simulink model "REBEC2A_Remote"  (R2022b)
settings: Solver=VariableStepAuto  StartTime=0.0  StopTime=inf  FixedStep=0.001  RelTol=1e-3
InitFcn:
  | Remote = ihm_control;
  | import net.java.games.input.*;
StartFcn:
  | Throttle_Xbox = 'REBEC2A_Remote/Throttle_Xbox';
  | event_Throttle_Xbox = 'PostOutputs';
  | listener_Throttle_Xbox = @(app, event_Throttle_Xbox) updateGUI(Remote);
  | Throttle_Xbox_exec = add_exec_event_listener(Throttle_Xbox, event_Throttle_Xbox, listener_Throttle_Xbox);
  | 
  | Steering_Xbox = 'REBEC2A_Remote/Steering_Xbox';
  | event_Steering_Xbox = 'PostOutputs';
  | listener_Steering_Xbox = @(app, event_Steering_Xbox) updateGUI(Remote);
  | Steering_Xbox_exec = add_exec_event_listener(Steering_Xbox, event_Steering_Xbox, listener_Steering_Xbox);
  | 
  | Steering_IA = 'REBEC2A_Remote/Steering_IA';
  | event_Steering_IA = 'PostOutputs';
  | listener_Steering_IA = @(app, event_Steering_IA) updateGUI(Remote);
  | Steering_IA_exec = add_exec_event_listener(Steering_IA, event_Steering_IA, listener_Steering_IA);
  | 
  | Throttle_IA = 'REBEC2A_Remote/Throttle_IA';
  | event_Throttle_IA = 'PostOutputs';
  | listener_Throttle_IA = @(app, event_Throttle_IA) updateGUI(Remote);
  | Throttle_IA_exec = add_exec_event_listener(Throttle_IA, event_Throttle_IA, listener_Throttle_IA);
  | 
  | Steering_G920 = 'REBEC2A_Remote/Steering_G920';
  | event_Steering_G920 = 'PostOutputs';
  | listener_Steering_G920 = @(app, event_Steering_G920) updateGUI(Remote);
  | Steering_G920_exec = add_exec_event_listener(Steering_G920, event_Steering_G920, listener_Steering_G920);
  | 
  | Throttle_G920 = 'REBEC2A_Remote/Throttle_G920';
  | event_Throttle_G920 = 'PostOutputs';
  | listener_Throttle_G920 = @(app, event_Throttle_G920) updateGUI(Remote);
  | Throttle_G920_exec = add_exec_event_listener(Throttle_G920, event_Throttle_G920, listener_Throttle_G920);
  | 
  | ButtonA_G920 = 'REBEC2A_Remote/ButtonA_G920';
  | event_ButtonA_G920 = 'PostOutputs';
  | listener_ButtonA_G920 = @(app, event_ButtonA_G920) updateGUI(Remote);
  | ButtonA_G920_exec = add_exec_event_listener(ButtonA_G920, event_ButtonA_G920, listener_ButtonA_G920);
StopFcn:
  | close all force;
undefined symbols (not defined in the file or in its folder): DiscIntNeverNeededParam
libraries: simulink x2, vrlib x1
settings Model: SimulationMode=accelerator  Creator=Mathias Voigt  LastModifiedBy=Xen
settings SolverCC: AlgebraicLoopSolver=TrustRegion
settings DebuggingCC: UnconnectedInputMsg=warning  UnconnectedOutputMsg=warning  UnconnectedLineMsg=warning  SFMachineParentedDataDiag=warning
settings ModelReferenceCC: EnableRefExpFcnMdlSchedulingChecks=on
settings SFSimCC: CustomCodeUndefinedFunction=UseInterfaceOnly

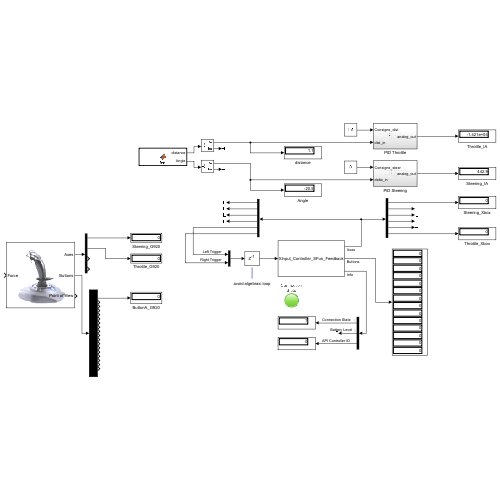
[thumbnail: Simulink's stored preview of the top-level diagram]
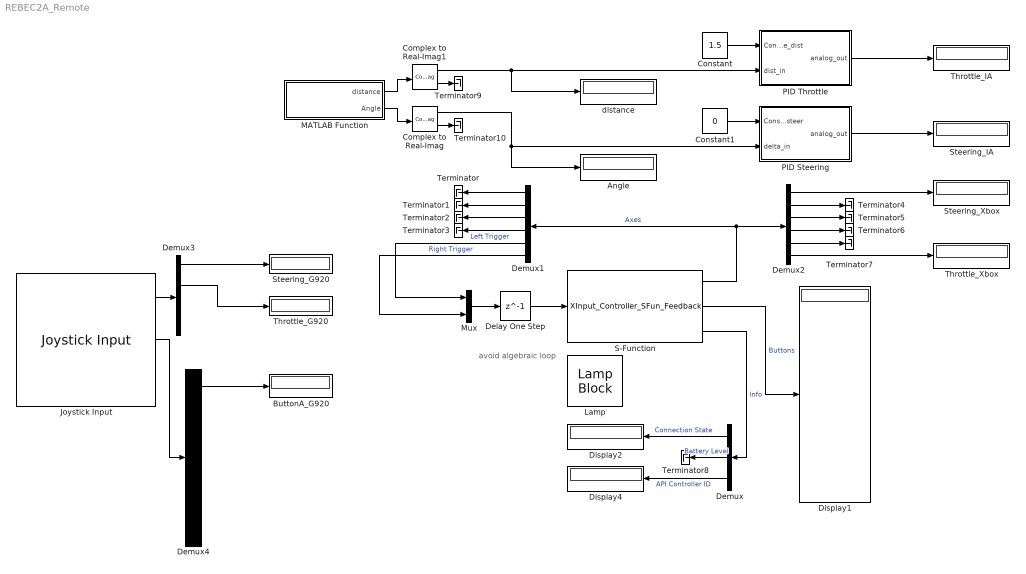
== system REBEC2A_Remote ==
  note: avoid algebraic loop
  Angle : Display
  ButtonA_G920 : Display
  Complex to Real-Imag : ComplexToRealImag
  Complex to Real-Imag1 : ComplexToRealImag
  Constant : Constant  Value=1.5
  Constant1 : Constant  Value=0
  Delay One Step : Delay  DelayLength=1
  Demux : Demux  Outputs=3
  Demux1 : Demux  Outputs=6
  Demux2 : Demux  Outputs=6
  Demux3 : Demux
  Demux4 : Demux  Outputs=18
  Display1 : Display
  Display2 : Display
  Display4 : Display
  Joystick Input : vrlib/Joystick Input  joyid=1  adjustports=on  forcefeed=on
  Lamp : LampBlock
  MATLAB Function : MATLAB Function  TreatAsAtomicUnit=on
  Mux : Mux  Inputs=2
  PID Steering : Subsystem
  PID Throttle : Subsystem
  S-Function : S-Function  FunctionName=XInput_Controller_SFun_Feedback  Parameters=1  SFunctionDeploymentMode=off  EnableBusSupport=off
  Steering_G920 : Display
  Steering_IA : Display
  Steering_Xbox : Display
  Terminator{,1..10} (11 alike) : Terminator
  Throttle_G920 : Display
  Throttle_IA : Display
  Throttle_Xbox : Display
  distance : Display
  wires:
  S-Function/2 -> Display1/1  "Buttons"
  S-Function/1 -> Demux1/1, Demux2/1  "Axes"
  Demux/1 -> Display2/1  "Connection State"
  Demux/3 -> Display4/1  "API Controller ID"
  S-Function/3 -> Demux/1  "Info"
  Delay One Step/1 -> S-Function/1
  Mux/1 -> Delay One Step/1
  Demux1/6 -> Mux/2  "Right Trigger"
  Demux1/5 -> Mux/1  "Left Trigger"
  Demux1/1 -> Terminator/1
  Demux1/2 -> Terminator1/1
  Demux1/3 -> Terminator2/1
  Demux1/4 -> Terminator3/1
  Demux2/6 -> Throttle_Xbox/1
  Constant/1 -> PID Throttle/1(Consigne_dist)
  Constant1/1 -> PID Steering/1(Consigne_steer)
  Demux2/1 -> Steering_Xbox/1
  Demux2/2 -> Terminator4/1
  Demux2/3 -> Terminator5/1
  Demux2/4 -> Terminator6/1
  Demux2/5 -> Terminator7/1
  Demux/2 -> Terminator8/1  "Battery Level"
  PID Throttle/1(analog_out) -> Throttle_IA/1
  PID Steering/1(analog_out) -> Steering_IA/1
  Complex to Real-Imag1/2 -> Terminator9/1
  Complex to Real-Imag/2 -> Terminator10/1
  MATLAB Function/1(distance) -> Complex to Real-Imag1/1
  MATLAB Function/2(Angle) -> Complex to Real-Imag/1
  Complex to Real-Imag1/1 -> distance/1, PID Throttle/2(dist_in)
  Complex to Real-Imag/1 -> Angle/1, PID Steering/2(delta_in)
  Joystick Input/1 -> Demux3/1
  Demux3/1 -> Steering_G920/1
  Demux3/2 -> Throttle_G920/1
  Joystick Input/2 -> Demux4/1
  Demux4/1 -> ButtonA_G920/1

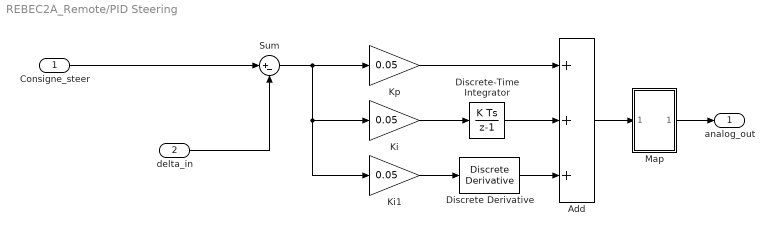
== system REBEC2A_Remote/PID Steering ==
  Consigne_steer : Inport
  delta_in : Inport  Port=2
  Add : Sum  Inputs=+++
  Discrete Derivative : simulink/Discrete/Discrete Derivative  gainval=1.0  ICPrevScaledInput=0.0  OutMin=[]  OutMax=[]  OutDataType=fixdt(1, 16)  OutScaling=2^-10  DoSatur=off
  Discrete-Time Integrator : DiscreteIntegrator  SampleTime=-1  ICPrevOutput=DiscIntNeverNeededParam  ICPrevScaledInput=DiscIntNeverNeededParam
  Ki : Gain  Gain=0.05
  Ki1 : Gain  Gain=0.05
  Kp : Gain  Gain=0.05
  Map : Subsystem
  Sum : Sum  Inputs=|+-
  analog_out : Outport
  wires:
  Kp/1 -> Add/1
  Sum/1 -> Ki1/1, Ki/1, Kp/1
  Ki1/1 -> Discrete Derivative/1
  Ki/1 -> Discrete-Time Integrator/1
  delta_in/1 -> Sum/2
  Consigne_steer/1 -> Sum/1
  Add/1 -> Map/1(In1)
  Map/1(Out1) -> analog_out/1
  Discrete-Time Integrator/1 -> Add/2
  Discrete Derivative/1 -> Add/3

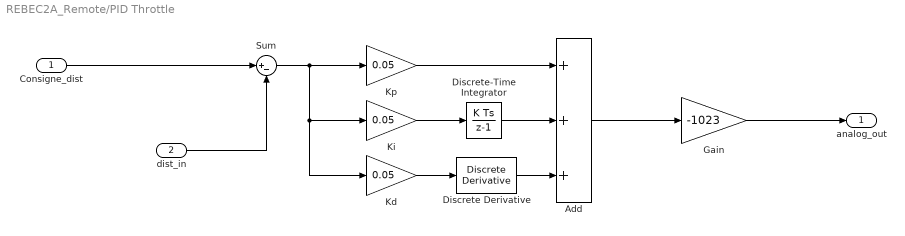
== system REBEC2A_Remote/PID Throttle ==
  Consigne_dist : Inport
  dist_in : Inport  Port=2
  Add : Sum  Inputs=+++
  Discrete Derivative : simulink/Discrete/Discrete Derivative  gainval=1.0  ICPrevScaledInput=0.0  OutMin=[]  OutMax=[]  OutDataType=fixdt(1, 16)  OutScaling=2^-10  DoSatur=off
  Discrete-Time Integrator : DiscreteIntegrator  SampleTime=-1  ICPrevOutput=DiscIntNeverNeededParam  ICPrevScaledInput=DiscIntNeverNeededParam
  Gain : Gain  Description=To fine tune  Gain=-1023
  Kd : Gain  Gain=0.05
  Ki : Gain  Gain=0.05
  Kp : Gain  Gain=0.05
  Sum : Sum  Inputs=|+-
  analog_out : Outport
  wires:
  Add/1 -> Gain/1
  Discrete Derivative/1 -> Add/3
  Kp/1 -> Add/1
  Sum/1 -> Kd/1, Ki/1, Kp/1
  Ki/1 -> Discrete-Time Integrator/1
  Discrete-Time Integrator/1 -> Add/2
  dist_in/1 -> Sum/2
  Gain/1 -> analog_out/1
  Consigne_dist/1 -> Sum/1
  Kd/1 -> Discrete Derivative/1

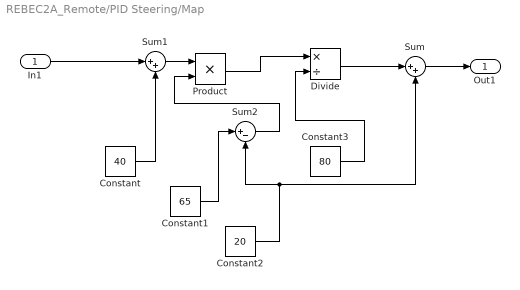
== system REBEC2A_Remote/PID Steering/Map ==
  In1 : Inport
  Constant : Constant  Value=40
  Constant1 : Constant  Value=65
  Constant2 : Constant  Value=20
  Constant3 : Constant  Value=80
  Divide : Product  Inputs=*/
  Product : Product
  Sum : Sum  Inputs=|++
  Sum1 : Sum  Inputs=|++
  Sum2 : Sum  Inputs=|+-
  Out1 : Outport
  wires:
  Constant1/1 -> Sum2/1
  Constant/1 -> Sum1/2
  Product/1 -> Divide/1
  Constant3/1 -> Divide/2
  Sum1/1 -> Product/1
  Constant2/1 -> Sum/2, Sum2/2
  Sum2/1 -> Product/2
  Divide/1 -> Sum/1
  In1/1 -> Sum1/1
  Sum/1 -> Out1/1

== matlab function REBEC2A_Remote/MATLAB Function ==
  data: distance output; Angle output
function [distance, Angle] = fcn()
    out1 = fileread("ImRec\distance.txt");
    out2 = fileread("ImRec\steering.txt");
    distance = str2double(out1);
    Angle = str2double(out2);
end
